simulink model "gm_sampleModel1667_sub"  (R2023a)
settings: Solver=VariableStepAuto  StartTime=0.0  StopTime=10.0  RelTol=1e-3
libraries: hdlsllib x1, simulink x1
settings Model: Creator=user1  LastModifiedBy=user1
settings OptimizationCC: BlockReduction=off  ConditionallyExecuteInputs=off
settings DebuggingCC: InheritedTsInSrcMsg=none

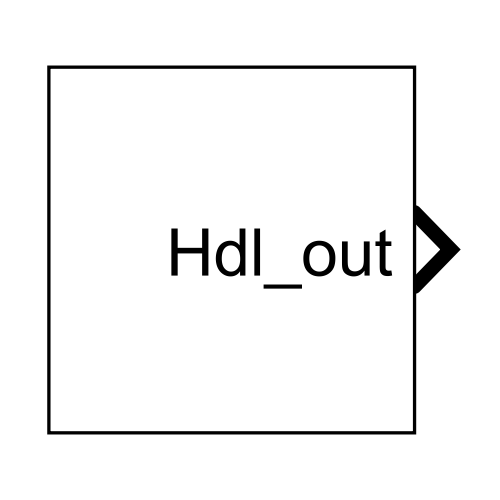
[thumbnail: Simulink's stored preview of the top-level diagram]
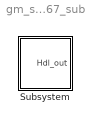
== system gm_sampleModel1667_sub ==
  Subsystem : Subsystem

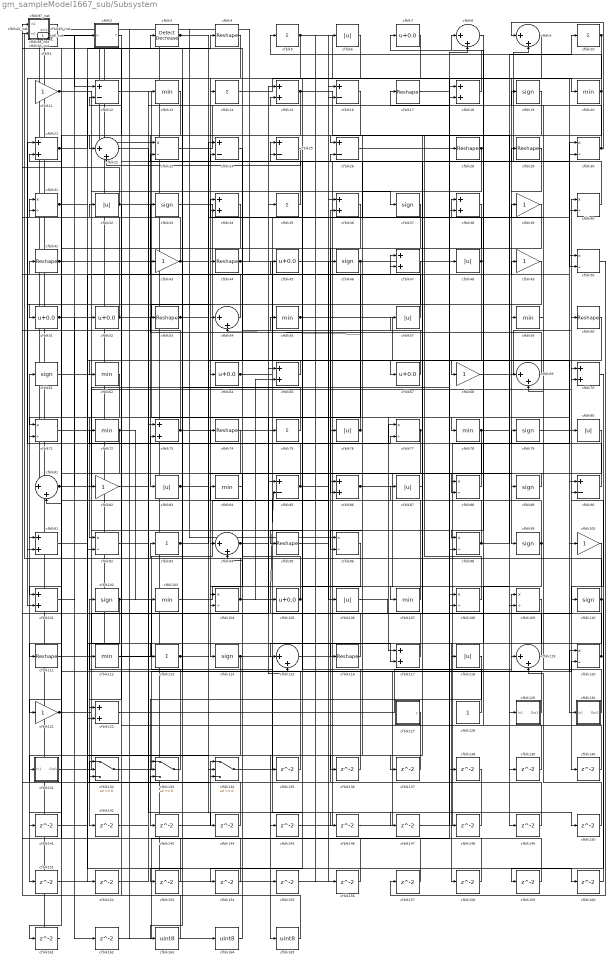
== system gm_sampleModel1667_sub/Subsystem ==
  cfblk1 : hdlsllib/Logic and Bit Operations/Bit Shift  mode=Shift Left Logical  N=0
  cfblk{5,10,14,35,75,93,113} (7 alike) : Sum  Inputs=+  OutDataTypeStr=uint8
  cfblk{11,39,43,49,68,82,100,121} (8 alike) : Gain  OutDataTypeStr=uint8
  cfblk{15,18,21,34,36,38,47,65,70,73,86,91,101,117,122} (15 alike) : Sum  OutDataTypeStr=uint8
  cfblk{19,33,37,46,61,79,89,99,102,110,114} (11 alike) : Signum
  cfblk{13,20,55,59,62,72,78,84,103,107,112} (11 alike) : MinMax  OutDataTypeStr=uint8
  cfblk{23,30..31,40,50,71,77,88,92,96,98,104,108..109,120} (15 alike) : Product  Inputs=*/  OutDataTypeStr=uint8  RndMeth=Zero  SaturateOnIntegerOverflow=on
  cfblk{7,45,51..52,64,67,105} (7 alike) : Bias  Bias=0.0  SaturateOnIntegerOverflow=off
  cfblk{6,32,48,57,76,80,83,87,106,118} (10 alike) : Abs  OutDataTypeStr=uint8  SaturateOnIntegerOverflow=off
  cfblk{4,17,28..29,41,44,53,60,74,95,111,116} (12 alike) : Reshape
  cfblk{8..9,22,54,69,81,94,115,119} (9 alike) : Sum  Inputs=|++  OutDataTypeStr=uint8
  cfblk{12,16,24..26,85,90} (7 alike) : Sum  Inputs=+-  OutDataTypeStr=uint8
  cfblk127 : Subsystem  mask(Counter Free-Running){NumBits=double(16), tsamp=double(-1)}
      mask prompts: NumBits "Simulink:masks:NumberOfBits_MP"; tsamp "Simulink:masks:SampleTime_MP"
      mask help: Simulink:masks:CounterFreeRunning_MD
  cfblk128 : Constant  OutDataTypeStr=uint8  SampleTime=-1
  cfblk129 : Subsystem
  cfblk130 : Subsystem
  cfblk131 : Subsystem
  cfblk132 : Switch  OutDataTypeStr=uint8  SaturateOnIntegerOverflow=off  InputSameDT=off
  cfblk133 : Switch  OutDataTypeStr=uint8  SaturateOnIntegerOverflow=off  InputSameDT=off
  cfblk134 : Switch  OutDataTypeStr=uint8  SaturateOnIntegerOverflow=off  InputSameDT=off
  cfblk{135..162} (28 alike) : Delay  SampleTime=1
  cfblk163 : DataTypeConversion  OutDataTypeStr=uint8  SaturateOnIntegerOverflow=off  RndMeth=Floor
  cfblk164 : DataTypeConversion  OutDataTypeStr=uint8  SaturateOnIntegerOverflow=off  RndMeth=Floor
  cfblk165 : DataTypeConversion  OutDataTypeStr=uint8  SaturateOnIntegerOverflow=off  RndMeth=Floor
  cfblk2 : Subsystem  mask(Detect Rise Positive){vinit=double(0), InputProcessing=Elements as channels (sample based), OutDataTypeStr=uint8}
      mask prompts: vinit "Simulink:masks:InitialCondition_MP"; InputProcessing "Simulink:masks:InputProcessing_MP"; OutDataTypeStr "Simulink:masks:OutputDataType_MP"
      mask help: Simulink:masks:DetectRisePositive_MD
      mask init:
      | InputProcessing = 'Elements as channels (sample based)';
      | OutDataTypeStr = 'uint8';
      | vinit = double(0);
      mask TypeOptions InputProcessing: Simulink:masks:ColumnsAsChannelsFrameBased | Simulink:masks:ElementsAsChannelsSampleBased
      mask TypeOptions OutDataTypeStr: Simulink:masks:uint8 | Simulink:masks:boolean
      mask Display: fprintf('U > 0\n&  NOT\nU/z > 0')
  cfblk27_inst : Subsystem
  cfblk3 : simulink/Logic and Bit Operations/Detect Decrease  vinit=0.0  OutDataTypeStr=uint8
      settings: LibrarySourceBlock=|
      | hdlsllib/Logic and Bit
      | Operations/Detect
      | Decrease
  cfblk42_inst : Subsystem
  cfblk56_inst : Subsystem
  cfblk58_inst : Subsystem
  cfblk63_inst : Subsystem
  cfblk97_inst : Subsystem
  Hdl_out : Outport  OutDataTypeStr=uint8  SampleTime=1
  wires:
  cfblk1/1 -> cfblk12/1
  cfblk10/1 -> cfblk99/1, cfblk114/1
  cfblk100/1 -> cfblk140/1
  cfblk101/1 -> cfblk152/1
  cfblk102/1 -> cfblk47/1, cfblk142/1
  cfblk103/1 -> cfblk107/1
  cfblk104/1 -> cfblk85/2, cfblk65/2, cfblk27_inst/2(in2)
  cfblk105/1 -> cfblk24/2, cfblk84/1
  cfblk106/1 -> cfblk25/1
  cfblk107/1 -> cfblk42_inst/1(in1)
  cfblk108/1 -> cfblk26/1
  cfblk109/1 -> cfblk154/1
  cfblk11/1 -> cfblk37/1, cfblk117/2
  cfblk110/1 -> cfblk159/1, cfblk158/1, cfblk93/1
  cfblk111/1 -> cfblk102/1
  cfblk112/1 -> cfblk16/1
  cfblk113/1 -> cfblk120/2, Hdl_out/1
  cfblk114/1 -> cfblk151/1, cfblk150/1
  cfblk115/1 -> cfblk9/2
  cfblk116/1 -> cfblk25/2
  cfblk117/1 -> cfblk56_inst/1(in1)
  cfblk118/1 -> cfblk143/1
  cfblk119/1 -> cfblk61/1
  cfblk12/1 -> cfblk78/1
  cfblk120/1 -> cfblk79/1, cfblk40/1
  cfblk121/1 -> cfblk52/1, cfblk35/1
  cfblk122/1 -> cfblk109/1
  cfblk127/1(y) -> cfblk165/1
  cfblk128/1 -> cfblk105/1
  cfblk129/1(Out1) -> cfblk41/1
  cfblk13/1 -> cfblk83/1
  cfblk130/1(Out1) -> cfblk34/1
  cfblk131/1(Out1) -> cfblk13/1
  cfblk132/1 -> cfblk119/1
  cfblk133/1 -> cfblk112/1
  cfblk134/1 -> cfblk70/1
  cfblk135/1 -> cfblk23/2
  cfblk136/1 -> cfblk85/1
  cfblk137/1 -> cfblk133/2
  cfblk138/1 -> cfblk133/3
  cfblk139/1 -> cfblk12/2
  cfblk14/1 -> cfblk20/1
  cfblk140/1 -> cfblk8/1
  cfblk141/1 -> cfblk134/1
  cfblk142/1 -> cfblk15/2
  cfblk143/1 -> cfblk134/3
  cfblk144/1 -> cfblk97_inst/2(in2)
  cfblk145/1 -> cfblk38/1
  cfblk146/1 -> cfblk120/1
  cfblk147/1 -> cfblk40/2
  cfblk148/1 -> cfblk91/1
  cfblk149/1 -> cfblk36/2
  cfblk15/1 -> cfblk81/2, cfblk129/1(In1)
  cfblk150/1 -> cfblk119/2
  cfblk151/1 -> cfblk77/2
  cfblk152/1 -> cfblk73/1
  cfblk153/1 -> cfblk132/1
  cfblk154/1 -> cfblk56_inst/2(in2)
  cfblk155/1 -> cfblk16/2
  cfblk156/1 -> cfblk71/2
  cfblk157/1 -> cfblk31/1
  cfblk158/1 -> cfblk132/3
  cfblk159/1 -> cfblk94/2
  cfblk16/1 -> cfblk51/1
  cfblk160/1 -> cfblk90/2
  cfblk161/1 -> cfblk1/1
  cfblk162/1 -> cfblk18/2
  cfblk163/1 -> cfblk32/1
  cfblk164/1 -> cfblk74/1
  cfblk165/1 -> cfblk58_inst/1(in1)
  cfblk17/1 -> cfblk108/1
  cfblk18/1 -> cfblk7/1
  cfblk19/1 -> cfblk137/1
  cfblk2/1(Y) -> cfblk22/1
  cfblk20/1 -> cfblk86/2, cfblk5/1
  cfblk21/1 -> cfblk4/1, cfblk116/1
  cfblk22/1 -> cfblk144/1
  cfblk23/1 -> cfblk15/1
  cfblk24/1 -> cfblk64/1
  cfblk25/1 -> cfblk22/2
  cfblk26/1 -> cfblk148/1
  cfblk27_inst/1(out1) -> cfblk81/1, cfblk11/1
  cfblk28/1 -> cfblk98/1, cfblk96/2, cfblk88/2
  cfblk29/1 -> cfblk59/1
  cfblk3/1 -> cfblk147/1, cfblk146/1
  cfblk30/1 -> cfblk9/1, cfblk17/1
  cfblk31/1 -> cfblk134/2, cfblk160/1
  cfblk32/1 -> cfblk58_inst/2(in2), cfblk122/1, cfblk117/1
  cfblk33/1 -> cfblk80/1
  cfblk34/1 -> cfblk44/1
  cfblk35/1 -> cfblk24/1
  cfblk36/1 -> cfblk71/1
  cfblk37/1 -> cfblk86/1
  cfblk38/1 -> cfblk131/1(In1)
  cfblk39/1 -> cfblk136/1
  cfblk4/1 -> cfblk14/1
  cfblk40/1 -> cfblk97_inst/1(in1)
  cfblk41/1 -> cfblk90/1, cfblk115/2
  cfblk42_inst/1(out1) -> cfblk164/1, cfblk155/1
  cfblk43/1 -> cfblk21/2, cfblk39/1
  cfblk44/1 -> cfblk30/2, cfblk149/1, cfblk108/2
  cfblk45/1 -> cfblk106/1
  cfblk46/1 -> cfblk101/1, cfblk92/1
  cfblk47/1 -> cfblk141/1
  cfblk48/1 -> cfblk95/1, cfblk26/2, cfblk153/1
  cfblk49/1 -> cfblk91/2
  cfblk5/1 -> cfblk38/2, cfblk122/2, cfblk50/2, cfblk156/1
  cfblk50/1 -> cfblk157/1
  cfblk51/1 -> cfblk49/1, cfblk162/1
  cfblk52/1 -> cfblk54/1, cfblk42_inst/2(in2)
  cfblk53/1 -> cfblk76/1, cfblk67/1
  cfblk54/1 -> cfblk33/1
  cfblk55/1 -> cfblk139/1, cfblk100/1
  cfblk56_inst/1(out1) -> cfblk48/1
  cfblk57/1 -> cfblk63_inst/2(in2)
  cfblk58_inst/1(out1) -> cfblk96/1
  cfblk59/1 -> cfblk19/1
  cfblk6/1 -> cfblk101/2
  cfblk60/1 -> cfblk132/2
  cfblk61/1 -> cfblk94/1
  cfblk62/1 -> cfblk161/1
  cfblk63_inst/1(out1) -> cfblk75/1
  cfblk64/1 -> cfblk46/1, cfblk28/1
  cfblk65/1 -> cfblk62/1
  cfblk67/1 -> cfblk63_inst/1(in1)
  cfblk68/1 -> cfblk60/1
  cfblk69/1 -> cfblk53/1
  cfblk7/1 -> cfblk133/1
  cfblk70/1 -> cfblk110/1
  cfblk71/1 -> cfblk8/2
  cfblk72/1 -> cfblk92/2, cfblk103/1
  cfblk73/1 -> cfblk65/1, cfblk27_inst/1(in1), cfblk31/2
  cfblk74/1 -> cfblk163/1
  cfblk75/1 -> cfblk3/1
  cfblk76/1 -> cfblk54/2, cfblk45/1
  cfblk77/1 -> cfblk111/1, cfblk121/1
  cfblk78/1 -> cfblk69/1, cfblk104/2
  cfblk79/1 -> cfblk130/1(In1)
  cfblk8/1 -> cfblk68/1
  cfblk80/1 -> cfblk145/1
  cfblk81/1 -> cfblk70/2, cfblk6/1, cfblk2/1(U)
  cfblk82/1 -> cfblk29/1
  cfblk83/1 -> cfblk88/1, cfblk77/1
  cfblk84/1 -> cfblk104/1
  cfblk85/1 -> cfblk36/1, cfblk21/1, cfblk72/1
  cfblk86/1 -> cfblk89/1, cfblk138/1
  cfblk87/1 -> cfblk57/1
  cfblk88/1 -> cfblk55/1
  cfblk89/1 -> cfblk82/1
  cfblk9/1 -> cfblk135/1
  cfblk90/1 -> cfblk73/2
  cfblk91/1 -> cfblk113/1
  cfblk92/1 -> cfblk98/2
  cfblk93/1 -> cfblk43/1, cfblk30/1
  cfblk94/1 -> cfblk47/2, cfblk18/1, cfblk50/1
  cfblk95/1 -> cfblk109/2
  cfblk96/1 -> cfblk115/1
  cfblk97_inst/1(out1) -> cfblk23/1
  cfblk98/1 -> cfblk87/1, cfblk10/1
  cfblk99/1 -> cfblk69/2, cfblk34/2, cfblk118/1

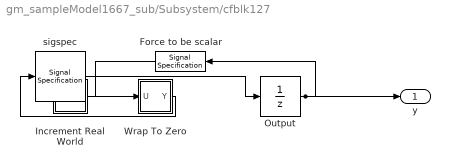
== system gm_sampleModel1667_sub/Subsystem/cfblk127 ==
  Force to be scalar : SignalSpecification  DisableCoverage=on  Dimensions=1
  Increment Real World : Subsystem  mask(Real World Value Increment){}
      mask help: Simulink:masks:RealWorldValueIncrement_MD
      mask Display: disp('V++')
  Output : UnitDelay  InitialCondition=0.0  SampleTime=tsamp  HasFrameUpgradeWarning=on
  Wrap To Zero : Subsystem  mask(Wrap To Zero){Threshold=double(65535)}
      mask prompts: Threshold "Simulink:masks:Threshold_MP"
      mask help: Simulink:masks:WrapToZero_MD
  sigspec : SignalSpecification  OutDataTypeStr=uint16  Dimensions=1
  y : Outport  SampleTime=1
  wires:
  Force to be scalar/1 -> Increment Real World/1(u)
  Increment Real World/1(y) -> Wrap To Zero/1(U)
  Output/1 -> Force to be scalar/1, y/1
  Wrap To Zero/1(Y) -> sigspec/1
  sigspec/1 -> Output/1

== system gm_sampleModel1667_sub/Subsystem/cfblk129 ==
  In1 : Inport  OutDataTypeStr=uint8  PortDimensions=1  SampleTime=1
  Out1 : Outport  SampleTime=1
  wires:
  In1/1 -> Out1/1

== system gm_sampleModel1667_sub/Subsystem/cfblk130 ==
  In1 : Inport  OutDataTypeStr=uint8  PortDimensions=1  SampleTime=1
  Out1 : Outport  SampleTime=1
  wires:
  In1/1 -> Out1/1

== system gm_sampleModel1667_sub/Subsystem/cfblk131 ==
  In1 : Inport  OutDataTypeStr=uint8  PortDimensions=1  SampleTime=1
  Out1 : Outport  SampleTime=1
  wires:
  In1/1 -> Out1/1

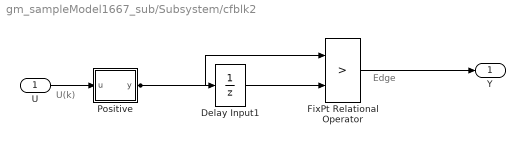
== system gm_sampleModel1667_sub/Subsystem/cfblk2 ==
  note: U(k)
  note: Edge
  U : Inport  OutDataTypeStr=uint8  SampleTime=1
  Delay Input1 : UnitDelay  Description=Store in Global RAM  DisableCoverage=on  InitialCondition=vinit  SampleTime=-1  HasFrameUpgradeWarning=on
  FixPt Relational Operator : RelationalOperator  Operator=>  OutDataTypeStr=fixdt(0, 8)  ZeroCross=off  InputSameDT=off
  Positive : Subsystem  mask(Compare To Zero){relop=>, OutDataTypeStr=boolean, ZeroCross=off}
      mask prompts: relop "Simulink:masks:Operator_MP"; OutDataTypeStr "Simulink:masks:OutputDataType_MP"; ZeroCross "Simulink:masks:EnableZerocrossingDetection_MP"
      mask help: Simulink:masks:CompareToZero_MD
      mask init:
      | OutDataTypeStr = 'boolean';
      | ZeroCross = 'off';
      | blkName = 'sampleModel1667_sub/Subsystem/cfblk2/Positive';
      | relop = '>';
      | setValue = 'boolean';
      mask TypeOptions relop: == | ~= | < | <= | >= | >
      mask TypeOptions OutDataTypeStr: Simulink:masks:uint8 | Simulink:masks:boolean
      mask Callback ZeroCross: sl('zeroCrossEnable', gcbh);
      mask Display: disp([relop,' 0'])
  Y : Outport  SampleTime=1
  wires:
  U/1 -> Positive/1(u)
  Delay Input1/1 -> FixPt Relational Operator/2
  FixPt Relational Operator/1 -> Y/1
  Positive/1(y) -> FixPt Relational Operator/1, Delay Input1/1

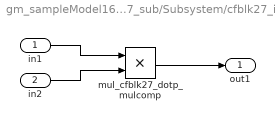
== system gm_sampleModel1667_sub/Subsystem/cfblk27_inst ==
  in1 : Inport  OutDataTypeStr=uint8  SampleTime=1
  in2 : Inport  Port=2  OutDataTypeStr=uint8  SampleTime=1
  mul_cfblk27_dotp_mulcomp : Product  Inputs=**  OutDataTypeStr=uint8  SampleTime=1
  out1 : Outport  OutDataTypeStr=uint8  SampleTime=1
  wires:
  in1/1 -> mul_cfblk27_dotp_mulcomp/1
  in2/1 -> mul_cfblk27_dotp_mulcomp/2
  mul_cfblk27_dotp_mulcomp/1 -> out1/1

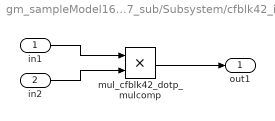
== system gm_sampleModel1667_sub/Subsystem/cfblk42_inst ==
  in1 : Inport  OutDataTypeStr=uint8  SampleTime=1
  in2 : Inport  Port=2  OutDataTypeStr=uint8  SampleTime=1
  mul_cfblk42_dotp_mulcomp : Product  Inputs=**  OutDataTypeStr=uint8  SampleTime=1
  out1 : Outport  OutDataTypeStr=uint8  SampleTime=1
  wires:
  in1/1 -> mul_cfblk42_dotp_mulcomp/1
  in2/1 -> mul_cfblk42_dotp_mulcomp/2
  mul_cfblk42_dotp_mulcomp/1 -> out1/1

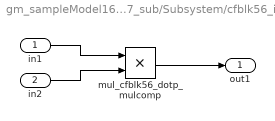
== system gm_sampleModel1667_sub/Subsystem/cfblk56_inst ==
  in1 : Inport  OutDataTypeStr=uint8  SampleTime=1
  in2 : Inport  Port=2  OutDataTypeStr=uint8  SampleTime=1
  mul_cfblk56_dotp_mulcomp : Product  Inputs=**  OutDataTypeStr=uint8  SampleTime=1
  out1 : Outport  OutDataTypeStr=uint8  SampleTime=1
  wires:
  in1/1 -> mul_cfblk56_dotp_mulcomp/1
  in2/1 -> mul_cfblk56_dotp_mulcomp/2
  mul_cfblk56_dotp_mulcomp/1 -> out1/1

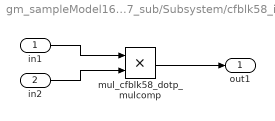
== system gm_sampleModel1667_sub/Subsystem/cfblk58_inst ==
  in1 : Inport  OutDataTypeStr=uint8  SampleTime=1
  in2 : Inport  Port=2  OutDataTypeStr=uint8  SampleTime=1
  mul_cfblk58_dotp_mulcomp : Product  Inputs=**  OutDataTypeStr=uint8  SampleTime=1
  out1 : Outport  OutDataTypeStr=uint8  SampleTime=1
  wires:
  in1/1 -> mul_cfblk58_dotp_mulcomp/1
  in2/1 -> mul_cfblk58_dotp_mulcomp/2
  mul_cfblk58_dotp_mulcomp/1 -> out1/1

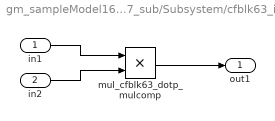
== system gm_sampleModel1667_sub/Subsystem/cfblk63_inst ==
  in1 : Inport  OutDataTypeStr=uint8  SampleTime=1
  in2 : Inport  Port=2  OutDataTypeStr=uint8  SampleTime=1
  mul_cfblk63_dotp_mulcomp : Product  Inputs=**  OutDataTypeStr=uint8  SampleTime=1
  out1 : Outport  OutDataTypeStr=uint8  SampleTime=1
  wires:
  in1/1 -> mul_cfblk63_dotp_mulcomp/1
  in2/1 -> mul_cfblk63_dotp_mulcomp/2
  mul_cfblk63_dotp_mulcomp/1 -> out1/1

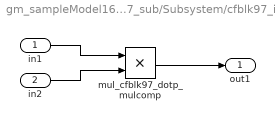
== system gm_sampleModel1667_sub/Subsystem/cfblk97_inst ==
  in1 : Inport  OutDataTypeStr=uint8  SampleTime=1
  in2 : Inport  Port=2  OutDataTypeStr=uint8  SampleTime=1
  mul_cfblk97_dotp_mulcomp : Product  Inputs=**  OutDataTypeStr=uint8  SampleTime=1
  out1 : Outport  OutDataTypeStr=uint8  SampleTime=1
  wires:
  in1/1 -> mul_cfblk97_dotp_mulcomp/1
  in2/1 -> mul_cfblk97_dotp_mulcomp/2
  mul_cfblk97_dotp_mulcomp/1 -> out1/1

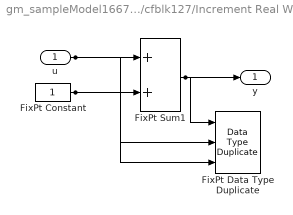
== system gm_sampleModel1667_sub/Subsystem/cfblk127/Increment Real World ==
  u : Inport  OutDataTypeStr=uint16  SampleTime=1
  FixPt Constant : Constant  DisableCoverage=on  OutDataTypeStr=Inherit: Inherit via back propagation  SampleTime=-1
  FixPt Data Type Duplicate : DataTypeDuplicate  DisableCoverage=on  NumInputPorts=3
  FixPt Sum1 : Sum  InputSameDT=on  OutDataTypeStr=Inherit: Inherit via back propagation  LockScale=on
  y : Outport  SampleTime=1
  wires:
  u/1 -> FixPt Sum1/1, FixPt Data Type Duplicate/2
  FixPt Constant/1 -> FixPt Sum1/2, FixPt Data Type Duplicate/3
  FixPt Sum1/1 -> FixPt Data Type Duplicate/1, y/1

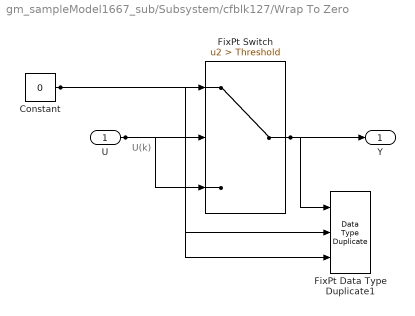
== system gm_sampleModel1667_sub/Subsystem/cfblk127/Wrap To Zero ==
  note: U(k)
  U : Inport  OutDataTypeStr=uint16  SampleTime=1
  Constant : Constant  DisableCoverage=on  Value=0  OutDataTypeStr=Inherit: Inherit via back propagation  SampleTime=-1
  FixPt Data Type Duplicate1 : DataTypeDuplicate  DisableCoverage=on  NumInputPorts=3
  FixPt Switch : Switch  Criteria=u2 > Threshold  Threshold=Threshold  OutDataTypeStr=Inherit: Inherit via back propagation  ZeroCross=off  SaturateOnIntegerOverflow=off  InputSameDT=off
  Y : Outport  SampleTime=1
  wires:
  U/1 -> FixPt Switch/3, FixPt Switch/2, FixPt Data Type Duplicate1/2
  Constant/1 -> FixPt Switch/1, FixPt Data Type Duplicate1/3
  FixPt Switch/1 -> FixPt Data Type Duplicate1/1, Y/1

== system gm_sampleModel1667_sub/Subsystem/cfblk2/Positive ==
  u : Inport  OutDataTypeStr=uint8  SampleTime=1
  Compare : RelationalOperator  Operator=>  OutDataTypeStr=boolean  ZeroCross=off
  Constant : Constant  DisableCoverage=on  Value=0  OutDataTypeStr=Inherit: Inherit via back propagation  SampleTime=-1  PreserveConstantTs=on
  y : Outport  SampleTime=1
  wires:
  u/1 -> Compare/1
  Compare/1 -> y/1
  Constant/1 -> Compare/2
